simulink model "Filtro_de_recepcao"  (R2013a)
settings: Solver=FixedStepDiscrete  StartTime=0.0  StopTime=10.0  RelTol=1e-3
values from neighbouring files (symbols this model uses):
  T = 1    [Variaveis.mat]
undefined symbols (not defined in the file or in its folder): St
libraries: dspsigops x2
settings Model: Creator=Élio  LastModifiedBy=Élio

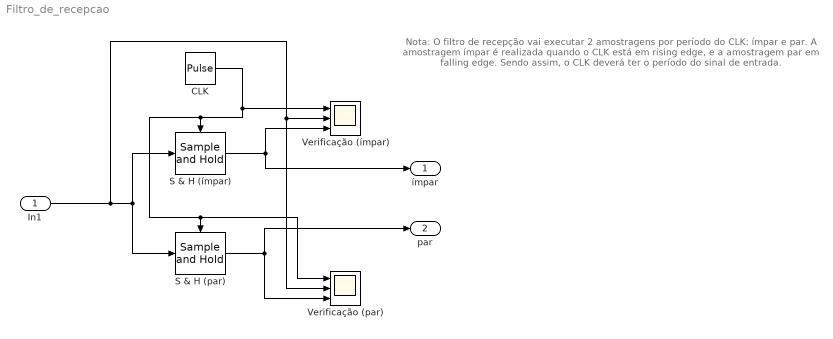
== system Filtro_de_recepcao ==
  note: Nota: O filtro de recepção vai executar 2 amostragens
      | por período do CLK: ímpar e par. A amostragem ímpar
      | é realizada quando o CLK está em rising edge, e a
      | amostragem par em falling edge. Sendo assim, o CLK
      | deverá ter o período do sinal de entrada.
  In1 : Inport
  CLK : DiscretePulseGenerator  PulseType=Time based  Period=2*T  PulseWidth=50  SampleTime=St
  "S & H (par) " : dspsigops/Sample and Hold  trig=Falling edge  initCond=0  latchinput=off
  "S & H (ímpar) " : dspsigops/Sample and Hold  trig=Rising edge  initCond=0  latchinput=off
  Verificação (par) : Scope  NumInputPorts=3
      settings: YMin=-5~-5~-5  YMax=5~5~5
  Verificação (ímpar) : Scope  NumInputPorts=3
      settings: YMin=-5~-5~-5  YMax=5~5~5
  ímpar : Outport
  par : Outport  Port=2
  wires:
  CLK/1 -> Verificação (ímpar)/1, Verificação (par)/1, "S & H (par) "/Trigger, "S & H (ímpar) "/Trigger
  In1/1 -> Verificação (ímpar)/2, Verificação (par)/2, "S & H (ímpar) "/1, "S & H (par) "/1
  "S & H (par) "/1 -> par/1, Verificação (par)/3
  "S & H (ímpar) "/1 -> ímpar/1, Verificação (ímpar)/3
